simulink model "Sudarshan_1_lab_8"  (R2022b)
settings: Solver=VariableStepAuto  StartTime=0.0  StopTime=0.01  MaxStep=1e-5  RelTol=1e-3
libraries: dspsrcs4 x1
settings Model: Creator=year2  LastModifiedBy=year2

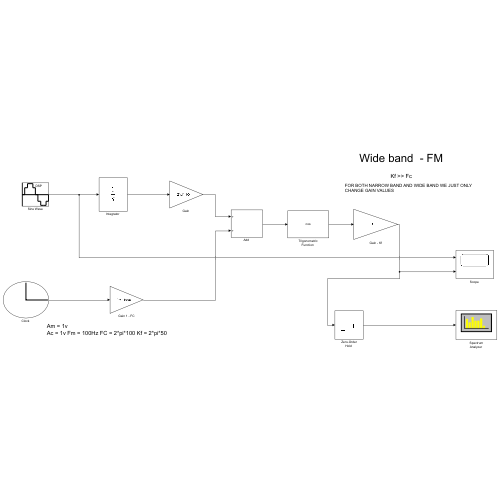
[thumbnail: Simulink's stored preview of the top-level diagram]
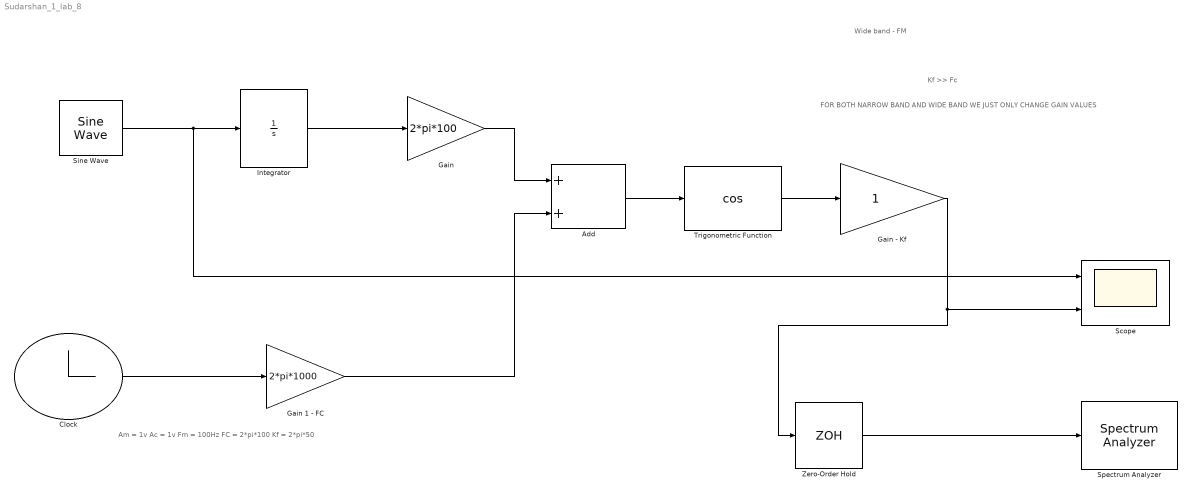
== system Sudarshan_1_lab_8 ==
  note: FOR BOTH NARROW BAND AND WIDE BAND WE JUST ONLY
      | CHANGE GAIN VALUES
  note: Kf >> Fc
  note: Am = 1v
      | Ac = 1v Fm = 100Hz FC = 2*pi*100 Kf = 2*pi*50
  note: Wide band - FM
  "Add " : Sum
  "Clock " : Clock
  "Gain " : Gain  Gain=2*pi*100
  Gain - Kf : Gain
  Gain 1 - FC : Gain  Gain=2*pi*1000
  "Integrator " : Integrator
  "Scope " : Scope  NumInputPorts=2
  Sine Wave : dspsrcs4/Sine Wave  Amplitude=1  Frequency=2*pi*100  Phase=0  SampleMode=Discrete  OutComplex=Real  CompMethod=Trigonometric fcn  TableSize=Speed  SampleTime=1/10000  SamplesPerFrame=1  ResetState=Restart at time zero  OutputFrames=off  dataType=double  wordLen=16  udDataType=sfix(16)  fracBitsMode=Best precision  numFracBits=15  OutDataTypeStr=double  LastOutDataTypeStr=double
  "Spectrum Analyzer " : SpectrumAnalyzer
  "Trigonometric Function " : Trigonometry  Operator=cos
  "Zero-Order Hold " : ZeroOrderHold  SampleTime=-1
  wires:
  Sine Wave/1 -> "Scope "/1, "Integrator "/1
  "Integrator "/1 -> "Gain "/1
  "Gain "/1 -> "Add "/1
  "Add "/1 -> "Trigonometric Function "/1
  "Trigonometric Function "/1 -> Gain - Kf/1
  Gain - Kf/1 -> "Zero-Order Hold "/1, "Scope "/2
  "Zero-Order Hold "/1 -> "Spectrum Analyzer "/1
  Gain 1 - FC/1 -> "Add "/2
  "Clock "/1 -> Gain 1 - FC/1
